simulink model "ModelPD"  (R2013b)
settings: Solver=ode45  StartTime=0.0  StopTime=50  RelTol=1e-3
values from neighbouring files (symbols this model uses):
  D = xopt(3)    [Plant1delay.m]    (also in Plant2.m; Plant2delay.m; Plant3.m; Plant4.m)
  denum = [T1(i) 1]    [Plant1delay.m]    (also in Plant2.m = [1 1 1]; Plant2delay.m = [T2(i)*T2(i) 2*T2(i) 1]; Plant3.m = [T3(i)*T3(i) T3(i)*T3(i)+2*T3 2*T3(i) 1 1]; Plant8.m = [1 3 3 1])
  N = xopt(4)    [Plant1delay.m]    (also in Plant2.m; Plant2delay.m; Plant3.m; Plant4.m)
  num = [1]    [Plant1delay.m]    (also in Plant2.m; Plant2delay.m; Plant3.m; Plant8.m = [-alfa8(i) 1])
  P = xopt(1)    [Plant1delay.m]    (also in Plant2.m; Plant2delay.m; Plant3.m; Plant4.m)
settings Model: Creator=stelmo  LastModifiedBy=stelmo

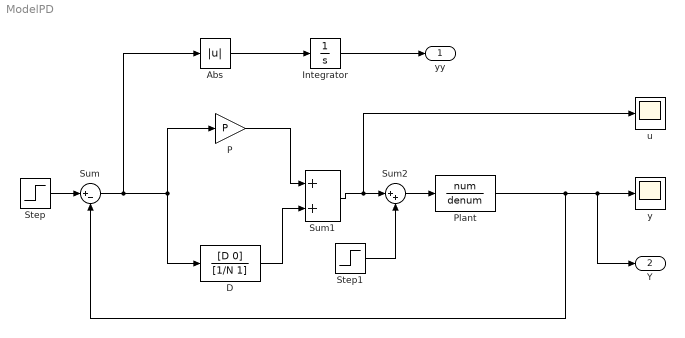
== system ModelPD ==
  Abs : Abs
  D : TransferFcn  Numerator=[D 0]  Denominator=[1/N 1]
  Integrator : Integrator
  P : Gain  Gain=P
  Plant : TransferFcn  Numerator=num  Denominator=denum
  Step : Step  SampleTime=0
  Step1 : Step  Time=5  After=-0.4  SampleTime=0
  Sum : Sum  Inputs=|+-
  Sum1 : Sum
  Sum2 : Sum  Inputs=|++
  u : Scope
  y : Scope
      settings: MaxDataPoints=50000000
  yy : Outport
  Y : Outport  Port=2
  wires:
  Step/1 -> Sum/1
  Sum/1 -> D/1, P/1, Abs/1
  Plant/1 -> Y/1, y/1, Sum/2
  Abs/1 -> Integrator/1
  Integrator/1 -> yy/1
  Sum1/1 -> Sum2/1, u/1
  P/1 -> Sum1/1
  Step1/1 -> Sum2/2
  Sum2/1 -> Plant/1
  D/1 -> Sum1/2
